simulink model "gravityGradient_test"  (R2018b)
settings: Solver=VariableStepAuto  StartTime=0.0  StopTime=0  RelTol=1e-3
values from neighbouring files (symbols this model uses):
  State = [reci;v;qd;w]    [gravityGradient_test_init.m]
  UTC = 137803367    [gravityGradient_test_init.m]
libraries: gravityGrad_Lib x1, time_Lib x1
settings Model: Creator=devantormey  LastModifiedBy=IvanMachuca

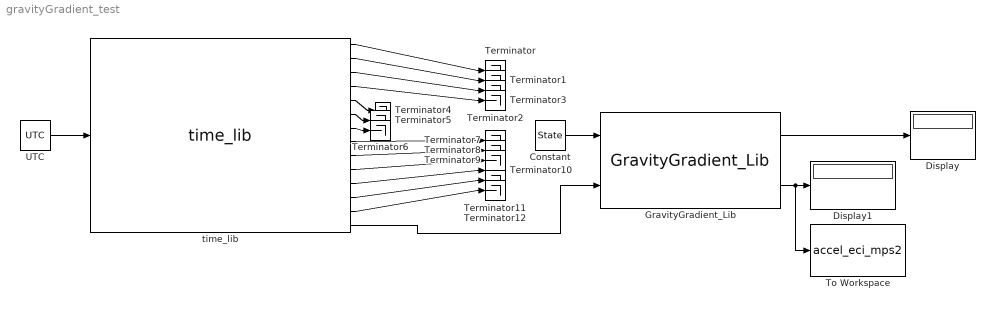
== system gravityGradient_test ==
  Constant : Constant  Value=State
  Display : Display
  Display1 : Display
  "GravityGradient_Lib " : gravityGrad_Lib/GravityGradient_Lib   SystemSampleTime=-1
  Terminator{,1..12} (13 alike) : Terminator
  To Workspace : ToWorkspace  VariableName=accel_eci_mps2  SampleTime=-1
      settings: Save2DSignal=2-D array (concatenate along first dimension)
  "UTC " : Constant  Value=UTC
  "time_lib " : time_Lib/time_lib    SystemSampleTime=-1
  wires:
  "GravityGradient_Lib "/2 -> To Workspace/1, Display1/1
  "GravityGradient_Lib "/1 -> Display/1
  Constant/1 -> "GravityGradient_Lib "/1
  "time_lib "/14 -> "GravityGradient_Lib "/2
  "time_lib "/1 -> Terminator/1
  "time_lib "/2 -> Terminator1/1
  "time_lib "/3 -> Terminator2/1
  "time_lib "/4 -> Terminator3/1
  "time_lib "/5 -> Terminator4/1
  "time_lib "/6 -> Terminator5/1
  "time_lib "/7 -> Terminator6/1
  "time_lib "/8 -> Terminator7/1
  "time_lib "/9 -> Terminator8/1
  "time_lib "/10 -> Terminator9/1
  "time_lib "/11 -> Terminator10/1
  "time_lib "/12 -> Terminator11/1
  "time_lib "/13 -> Terminator12/1
  "UTC "/1 -> "time_lib "/1
